simulink model "mpc_optimiert_test"  (R2019b)
settings: Solver=FixedStepAuto  StartTime=0.0  StopTime=10.0  FixedStep=1e-3  RelTol=1e-3
libraries: mpclib x1, cstblocks x1

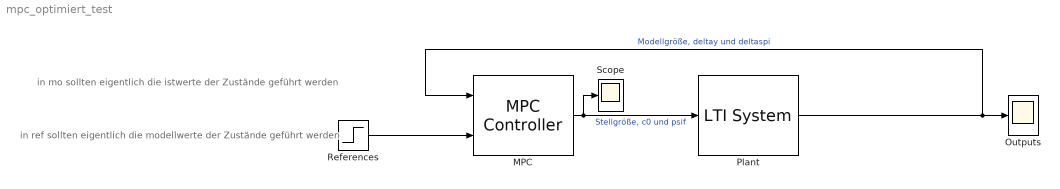
== system mpc_optimiert_test ==
  note: in ref sollten eigentlich die modellwerte der Zustände geführt werden
  note: in mo sollten eigentlich die istwerte der Zustände geführt werden
  MPC : mpclib/MPC Controller  SCDEnableBlockLinearizationSpecification=on  mpcobj=mpc1_C_1  is_multiple=0  enable_value=0  return_u0=off  updateMPCinCallerWorkspace=on  md_inport=off  mv_inport=off  uref_inport=off  return_cost=off  return_mvseq=off  return_qpstatus=off  return_xseq=off  return_state=off  return_ovseq=off  state_inport=off  umin_inport=off  umax_inport=off  ymin_inport=off  ymax_inport=off  cc_inport=off  ywt_inport=off  uwt_inport=off  duwt_inport=off  rhoeps_inport=off  pm_inport=off  MaximumP=10  HorizonChoice=FixedHorizon  n_ts=0.1  n_p=10  n_mv=2  n_md=0  n_ud=0  n_mo=2  n_uo=0  BlockDataType=double  SampleTimeInherited=off  switch_inport=off
  Outputs : Scope
  Plant : cstblocks/LTI System  sys=mpc1_G_1  IC=[]
  References : Step  Before=[0;0]  After=[1;1]
  Scope : Scope
  wires:
  References/1 -> MPC/2
  Plant/1 -> MPC/1, Outputs/1  "Modellgröße, deltay und deltaspi"
  MPC/1 -> Plant/1, Scope/1  "Stellgröße, c0 und psif"
